simulink model "Exp4_MODEL_EM"  (R2023b)
settings: Solver=ode3  StartTime=0  StopTime=Time(end)  FixedStep=1e-5  RelTol=1e-3
undefined symbols (not defined in the file): i_A, k_M, L_A, LT1D_R_LH, R_A, r_DG
settings Model: Creator=tunkarlu  LastModifiedBy=tunkarlu

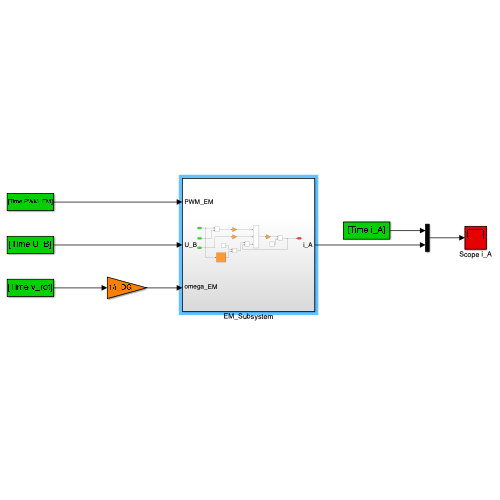
[thumbnail: Simulink's stored preview of the top-level diagram]
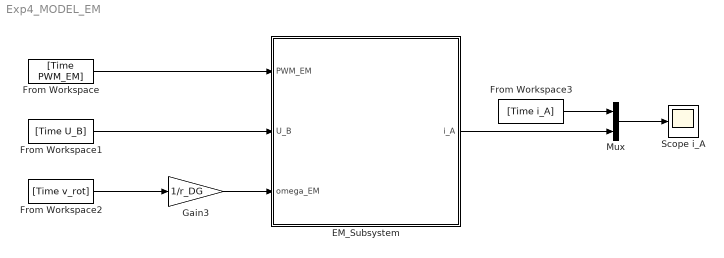
== system Exp4_MODEL_EM ==
  EM_Subsystem : Subsystem
  From Workspace : FromWorkspace  VariableName=[Time PWM_EM]
  From Workspace1 : FromWorkspace  VariableName=[Time U_B]
  From Workspace2 : FromWorkspace  VariableName=[Time v_rot]
  From Workspace3 : FromWorkspace  VariableName=[Time i_A]
  Gain3 : Gain  Gain=1/r_DG
  Mux : Mux  Inputs=2
  Scope i_A : Scope
  wires:
  From Workspace2/1 -> Gain3/1
  From Workspace/1 -> EM_Subsystem/1(PWM_EM)
  From Workspace1/1 -> EM_Subsystem/2(U_B)
  Gain3/1 -> EM_Subsystem/3(omega_EM)
  Mux/1 -> Scope i_A/1
  From Workspace3/1 -> Mux/1
  EM_Subsystem/1(i_A) -> Mux/2

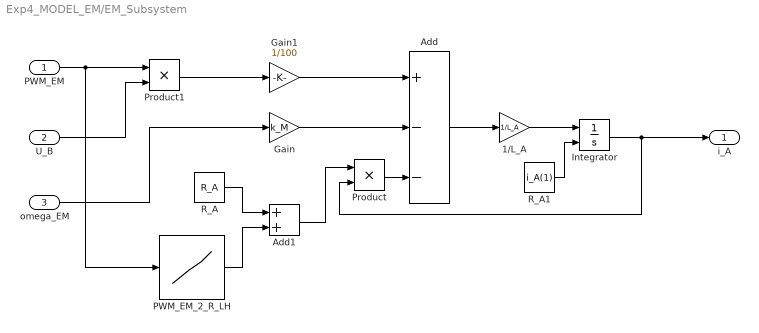
== system Exp4_MODEL_EM/EM_Subsystem ==
  PWM_EM : Inport
  U_B : Inport  Port=2
  omega_EM : Inport  Port=3
  1/L_A : Gain  Gain=1/L_A
  Add : Sum  Inputs=+--
  Add1 : Sum
  Gain : Gain  Gain=k_M
  Gain1 : Gain  Gain=1/100
  Integrator : Integrator  InitialConditionSource=external
  PWM_EM_2_R_LH : Lookup_n-D  NumberOfTableDimensions=1  BreakpointsForDimension1=LT1D_R_LH(1,:)  Table=LT1D_R_LH(2,:)  InternalRulePriority=Speed  RndMeth=Simplest
  Product : Product
  Product1 : Product
  R_A : Constant  Value=R_A
  R_A1 : Constant  Value=i_A(1)
  i_A : Outport
  wires:
  U_B/1 -> Product1/2
  omega_EM/1 -> Gain/1
  PWM_EM_2_R_LH/1 -> Add1/2
  R_A/1 -> Add1/1
  Add/1 -> 1/L_A/1
  Gain/1 -> Add/2
  Integrator/1 -> i_A/1, Product/2
  PWM_EM/1 -> PWM_EM_2_R_LH/1, Product1/1
  1/L_A/1 -> Integrator/1
  Product1/1 -> Gain1/1
  Add1/1 -> Product/1
  Product/1 -> Add/3
  Gain1/1 -> Add/1
  R_A1/1 -> Integrator/2
